simulink model "Block_ZU"  (R2022a)
settings: Solver=ode23tb  StartTime=0.0  StopTime=5  MaxStep=1e-4  RelTol=1e-5
undefined symbols (not defined in the file): DiscIntNeverNeededParam, ZU
libraries: simulink x1
settings Model: Creator=админ  LastModifiedBy=админ

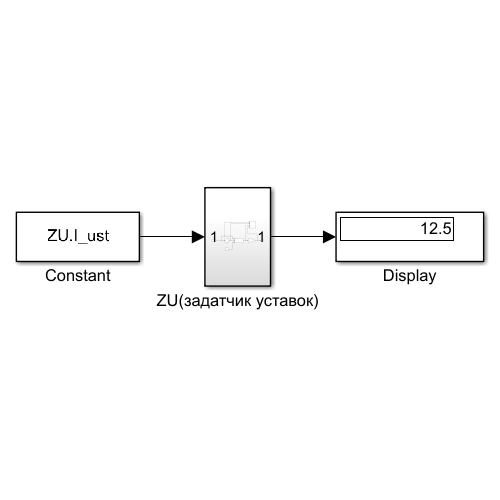
[thumbnail: Simulink's stored preview of the top-level diagram]
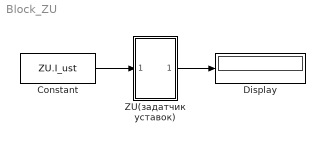
== system Block_ZU ==
  Constant : Constant  Value=ZU.I_ust
  Display : Display
  ZU(задатчик уставок) : Subsystem
  wires:
  Constant/1 -> ZU(задатчик уставок)/1(In1)
  ZU(задатчик уставок)/1(Out1) -> Display/1

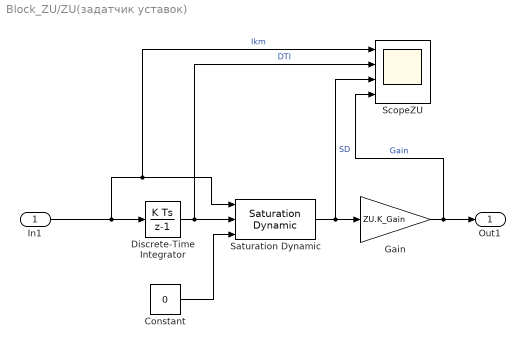
== system Block_ZU/ZU(задатчик уставок) ==
  In1 : Inport
  Constant : Constant  Value=0
  Discrete-Time Integrator : DiscreteIntegrator  gainval=0.5  SampleTime=1/100  ICPrevOutput=DiscIntNeverNeededParam  ICPrevScaledInput=DiscIntNeverNeededParam
  Gain : Gain  Gain=ZU.K_Gain
  Saturation Dynamic : simulink/Discontinuities/Saturation Dynamic  OutMin=[]  OutMax=[]  OutDataTypeStr=Inherit: Same as second input  OutDataType=fixdt(1, 16)  OutScaling=2^-10  DoSatur=off
  ScopeZU : Scope  NumInputPorts=4
  Out1 : Outport
  wires:
  Saturation Dynamic/1 -> ScopeZU/3, Gain/1  "SD"
  Discrete-Time Integrator/1 -> ScopeZU/2, Saturation Dynamic/2  "DTI"
  In1/1 -> ScopeZU/1, Saturation Dynamic/1, Discrete-Time Integrator/1  "Ikm"
  Constant/1 -> Saturation Dynamic/3
  Gain/1 -> ScopeZU/4, Out1/1  "Gain"
